simulink model "SkywalkerX8_AircraftModel"  (R2018a)
settings: Solver=FixedStepAuto  StartTime=0.0  StopTime=60  FixedStep=0.001  RelTol=1e-3
undefined symbols (not defined in the file): SkywalkerX8
settings Model: Creator=David  LastModifiedBy=David

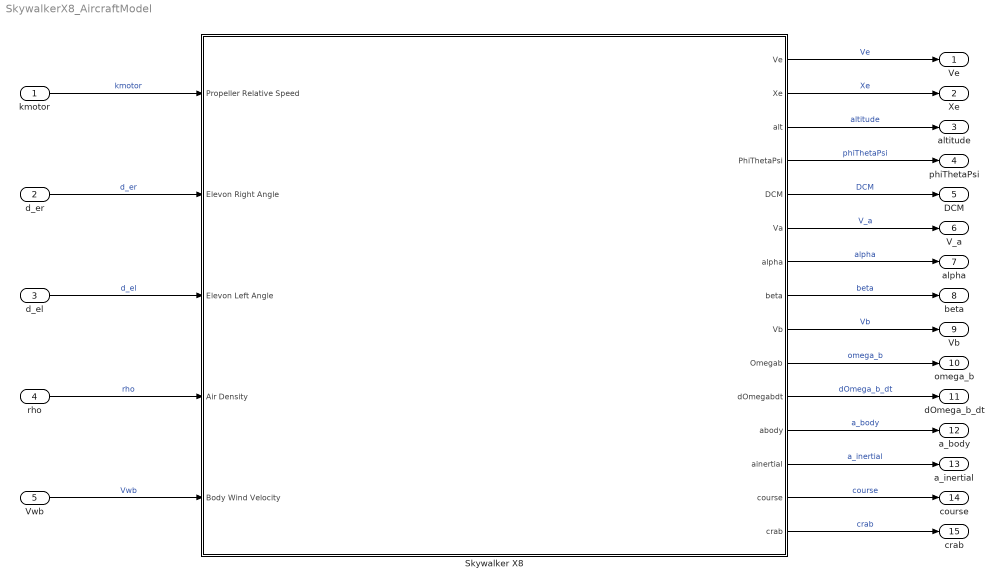
== system SkywalkerX8_AircraftModel ==
  kmotor : Inport
  d_er : Inport  Port=2
  d_el : Inport  Port=3
  rho : Inport  Port=4
  Vwb : Inport  Port=5  PortDimensions=[1, 3]
  Skywalker X8 : Subsystem  mask{PhiThetaPsi_init=[0, 0.194, 0], Xe_init=[0, 0, -100], Vb_init=[8.82, 0, 1.73], PhiThetaPsiDot_init=[0, 0, 0], Mass=SkywalkerX8.System.Mass, Inertia_Matrix=SkywalkerX8.System.InertiaTensor, g=SkywalkerX8.System.Gravity, CD=SkywalkerX8.Aerodynamics.CD, CY=SkywalkerX8.Aerodynamics.CY, CL=SkywalkerX8.Aerodynamics.CL, CI=SkywalkerX8.Aerodynamics.Cl, Cm=SkywalkerX8.Aerodynamics.Cm, Cn=SkywalkerX8.Aerodynamics.Cn, alpha_0=SkywalkerX8.Aerodynamics.alpha_0, M_trans=SkywalkerX8.Aerodynamics.M, Cmfp=SkywalkerX8.Aerodynamics.Cmfp, b=SkywalkerX8.Geometry.b, c=SkywalkerX8.Geometry.c, S=SkywalkerX8.Geometry.S, Sprop=SkywalkerX8.Propeller.Sprop, Cprop=SkywalkerX8.Propeller.Cprop, kmotor=SkywalkerX8.Propeller.kmotor, kOmega=SkywalkerX8.Propeller.kOmega, kTp=SkywalkerX8.Propeller.kTp}
      mask prompts: PhiThetaPsi_init "Inital roll, pitch and yaw angles [phi, theta, psi] (rad)"; Xe_init "Initial position in inertial frame [Xe, Ye, Ze] (m)"; Vb_init "Initial velocity in body frame [u, v, w] (m/s)"; PhiThetaPsiDot_init "Initial roll, pitch, yaw angular velocity d/dt[phi, theta, psi] (rad/s)"; Mass "System mass (kg)"; Inertia_Matrix "System Inertia Tensor [Jxx, Jxy, Jxz; Jyx, Jyy, Jyz; Jzx, Jzy, Jzz] (kg.m^2)"; g "Gravitational constant (m/s^2)"; CD "Drag force coefficient array, of multiple [1, alpha, alpha^2, cq/2Va, beta^2, beta, de^2]"; CY "Side force coefficient array, of multiple [1, beta, bp/2Va, br/2Va, da]"; CL "Lift force coefficient array, of multiple [1, alpha, cq/2Va, de]"; CI "Roll coefficient array, of multiple [1, beta, bp/2Va, br/2Va, da]"; Cm "Pitch coefficient array, of multiple [1, alpha, bq/2Va, de]"; Cn "Yaw coefficient array, of multiple [1, beta, bp/2Va, br/2Va, da]"; alpha_0 "Stall angle, alpha_0 (rad)"; M_trans "Transition rate, M"; Cmfp "Pitching moment flat plate coefficient, Cmfp"; b "Wing span, b (m)"; c "Mean aerodynamic chord, c (m)"; S "Wing area, S (m^2)"; Sprop "Propeller swept area, Sprop (m^2)"; Cprop "Propeller aerodynamic coefficient, Cprop"; kmotor "Motor constant, kmotor (m/s)"; kOmega "Motor angular velocity constant, kOmega (rad/s)"; kTp "Motor torque constant, kTp (Nm/(rad/s)^2)"
      mask DialogControl DescGroupVar Prompt: SkywalkerX8 Aircraft Model
      mask DialogControl DescTextVar Prompt: This block models the Skywalker X8 Blended Wing-Body aircraft. It takes in control inputs and environmental conditions and outputs the full 6 DoF response from the system.
      mask DialogControl Container4 Prompt: Initial Conditions
      mask DialogControl Container5 Prompt: System Characteristics
      mask DialogControl Container6 Prompt: Aerodynamic Coefficients
      mask DialogControl Container9 Prompt: Aerodynamic Stall Parameters
      mask DialogControl Container7 Prompt: Geometric Characteristics
      mask DialogControl Container10 Prompt: Propeller/Motor Characteristics
      mask Display:
      | image('C:\MATLAB\masters\icons\Skywalker Main Block Icon.png', 'center')
      | 
      | color('cyan')
      | 
      | port_label('input', 1, 'k_{motor} (Unitless)', 'texmode', 'on')
      | port_label('input', 2, '\delta_{er} (rad)', 'texmode', 'on')
      | port_label('input', 3, '\delta_{el} (rad)', 'texmode', 'on')
      | port_label('input', 4, '\rho (kg/m^3)', 'texmode', 'on')
      | port_label('input', 5, '{\bf V_w^b} (m/s)', 'texmode', 'on')
      | 
      | port_label('output', 1, '{\bf V_e} (m/s)', 'texmode', 'on')
      | port_label('output', 2, '{\bf X_e} (m)', 'texmode', 'on')
      | port_label('output', 3, 'Altitude (m)', 'texmode', 'on')
      | port_label('output', 4, '\phi \theta \psi (rad)', 'texmode', 'on')
      | port_label('output', 5, 'R_{inertial}^{body}', 'texmode', 'on')
      | port_label('output', 6, 'V_a (m/s)', 'texmode', 'on')
      | port_label('output', 7, 'alpha (rad)', 'texmode', 'on')
      | port_label('output', 8, 'beta (rad)', 'texmode', 'on')
      | port_label('output', 9, '{\bf V_b} (m/s)', 'texmode', 'on')
      | port_label('output', 10, '{\bf \omega_b} (rad/s)', 'texmode', 'on')
      | port_label('output', 11, '{\bf \delta\omega_b/\deltat} (rad/s^2)', 'texmode', 'on')
      | port_label('output', 12, '{\bf a_{body}} (m/s^2)', 'texmode', 'on')
      | port_label('output', 13, '{\bf a_{inertial}} (m/s^2)', 'texmode', 'on')
      | port_label('output', 14, '\chi (rad)', 'texmode', 'on')
      | port_label('output', 15, '\chi_c (rad)', 'texmode', 'on')
  Ve : Outport
  Xe : Outport  Port=2
  altitude : Outport  Port=3
  phiThetaPsi : Outport  Port=4
  DCM : Outport  Port=5
  V_a : Outport  Port=6
  alpha : Outport  Port=7
  beta : Outport  Port=8
  Vb : Outport  Port=9
  omega_b : Outport  Port=10
  dOmega_b_dt : Outport  Port=11
  a_body : Outport  Port=12
  a_inertial : Outport  Port=13
  course : Outport  Port=14
  crab : Outport  Port=15
  wires:
  kmotor/1 -> Skywalker X8/1(Propeller Relative Speed)  "kmotor"
  d_er/1 -> Skywalker X8/2(Elevon Right Angle)  "d_er"
  d_el/1 -> Skywalker X8/3(Elevon Left Angle)  "d_el"
  Skywalker X8/1(Ve) -> Ve/1  "Ve"
  Skywalker X8/2(Xe) -> Xe/1  "Xe"
  Skywalker X8/4(PhiThetaPsi) -> phiThetaPsi/1  "phiThetaPsi"
  Skywalker X8/9(Vb) -> Vb/1  "Vb"
  Skywalker X8/10(Omegab) -> omega_b/1  "omega_b"
  Skywalker X8/11(dOmegabdt) -> dOmega_b_dt/1  "dOmega_b_dt"
  Skywalker X8/12(abody) -> a_body/1  "a_body"
  Skywalker X8/13(ainertial) -> a_inertial/1  "a_inertial"
  rho/1 -> Skywalker X8/4(Air Density)  "rho"
  Vwb/1 -> Skywalker X8/5(Body Wind Velocity)  "Vwb"
  Skywalker X8/5(DCM) -> DCM/1  "DCM"
  Skywalker X8/6(Va) -> V_a/1  "V_a"
  Skywalker X8/3("alt ") -> altitude/1  "altitude"
  Skywalker X8/7(alpha) -> alpha/1  "alpha"
  Skywalker X8/8(beta) -> beta/1  "beta"
  Skywalker X8/14(course) -> course/1  "course"
  Skywalker X8/15(crab) -> crab/1  "crab"

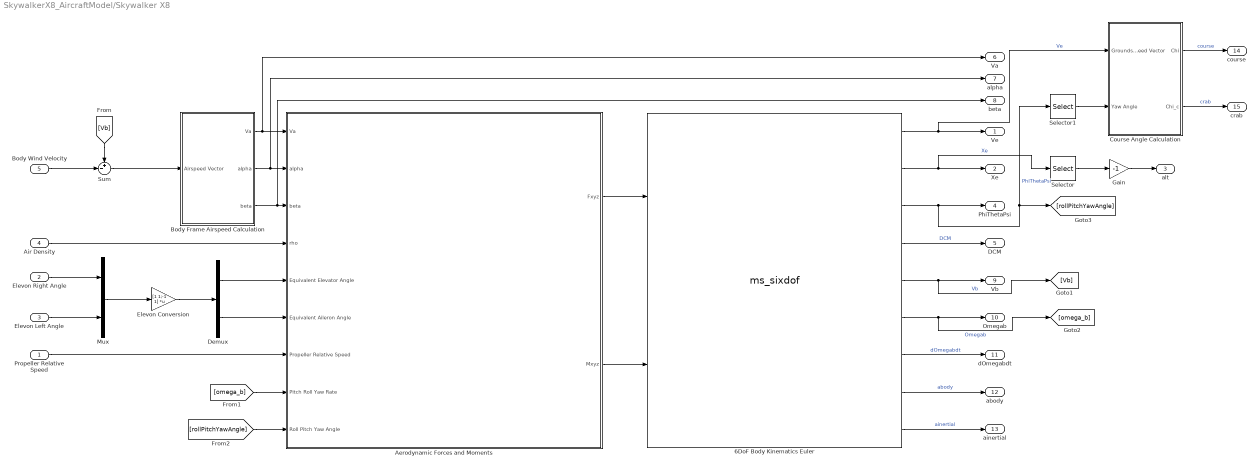
== system SkywalkerX8_AircraftModel/Skywalker X8 ==
  Propeller Relative Speed : Inport
  Elevon Right Angle : Inport  Port=2
  Elevon Left Angle : Inport  Port=3
  Air Density : Inport  Port=4
  Body Wind Velocity : Inport  Port=5
  6DoF Body Kinematics Euler : M-S-Function  FunctionName=ms_sixdof  Parameters=Xe_init, Vb_init, PhiThetaPsi_init, PhiThetaPsiDot_init, Mass, Inertia_Matrix  mask{PhiThetaPsi_init=PhiThetaPsi_init, Xe_init=Xe_init, Vb_init=Vb_init, PhiThetaPsiDot_init=PhiThetaPsiDot_init, Mass=Mass, Inertia_Matrix=Inertia_Matrix}
      mask prompts: PhiThetaPsi_init "Inital roll, pitch and yaw angles [phi, theta, psi] (rad)"; Xe_init "Initial position in inertial frame [Xe, Ye, Ze] (m)"; Vb_init "Initial velocity in body frame [u, v, w] (m/s)"; PhiThetaPsiDot_init "Initial roll, pitch, yaw angular velocity d/dt[phi, theta, psi] (rad/s)"; Mass "System mass (kg)"; Inertia_Matrix "System Inertia Tensor [Jxx, Jxy, Jxz; Jyx, Jyy, Jyz; Jzx, Jzy, Jzz] (kg.m^2)"
      mask DialogControl DescGroupVar Prompt: 6DoF Kinematics Model
      mask DialogControl DescTextVar Prompt: This block models the equations of motion for a 6DoF system in the body frame
      mask DialogControl Container4 Prompt: Initial Conditions
      mask DialogControl Container8 Prompt: System Parameters
      mask Display:
      | image('C:\MATLAB\masters\icons\6DoF Kinematics Block Icon.PNG', 'center')
      | 
      | port_label('input', 1, '{\bf F_{xyz}} (N)', 'texmode', 'on')
      | port_label('input', 2, '{\bf M_{xyz}} (Nm)', 'texmode', 'on')
      | 
      | port_label('output', 1, '{\bf V_e} (m/s)', 'texmode', 'on')
      | port_label('output', 2, '{\bf X_e} (m)', 'texmode', 'on')
      | port_label('output', 3, '\phi \theta \psi (rad)', 'texmode', 'on')
      | port_label('output', 4, 'R_{inertial}^{body}', 'texmode', 'on')
      | port_label('output', 5, '{\bf V_b} (m/s)', 'texmode', 'on')
      | port_label('output', 6, '{\bf \omega_b} (rad/s)', 'texmode', 'on')
      | port_label('output', 7, '{\bf \delta\omega_b/\deltat} (rad/s^2)', 'texmode', 'on')
      | port_label('output', 8, '{\bf a_{body}} (m/s^2)', 'texmode', 'on')
      | port_label('output', 9, '{\bf a_{inertial}} (m/s^2)', 'texmode', 'on')
  Aerodynamic Forces and Moments : Subsystem  mask{CD=CD, CY=CY, CL=CL, CI=CI, Cm=Cm, Cn=Cn, alpha_0=alpha_0, M_trans=M_trans, Cmfp=Cmfp, b=b, c=c, S=S, m=Mass, g=g, Sprop=Sprop, Cprop=Cprop, kmotor=kmotor, kOmega=kOmega, kTp=kTp}
      mask prompts: CD "Drag force coefficient array, of multiple [1, alpha, alpha^2, cq/2Va, beta^2, beta, de^2]"; CY "Side force coefficient array, of multiple [1, beta, bp/2Va, br/2Va, da]"; CL "Lift force coefficient array, of multiple [1, alpha, cq/2Va, de]"; CI "Roll coefficient array, of multiple [1, beta, bp/2Va, br/2Va, da]"; Cm "Pitch coefficient array, of multiple [1, alpha, bq/2Va, de]"; Cn "Yaw coefficient array, of multiple [1, beta, bp/2Va, br/2Va, da]"; alpha_0 "Stall angle, alpha_0 (rad)"; M_trans "Transition rate, M"; Cmfp "Pitching moment flat plate coefficient, Cmfp"; b "Wing span, b (m)"; c "Mean aerodynamic chord, c (m)"; S "Wing area, S (m^2)"; m "System mass, m (kg)"; g "Gravitational constant, g (m/s^2)"; Sprop "Propeller swept area, Sprop (m^2)"; Cprop "Propeller aerodynamic coefficient, Cprop"; kmotor "Motor constant, kmotor (m/s)"; kOmega "Motor angular velocity constant, kOmega (rad/s)"; kTp "Motor torque constant, kTp (Nm/(rad/s)^2)"
      mask DialogControl DescGroupVar Prompt: Aerodynamic Forces and Moments
      mask DialogControl DescTextVar Prompt: The purpose of this block is to calulate the aerodynamic forces and moments expeirenced by an aircraft exposed to a particular airflow, at a particular density, given a particular set of control surface inputs and motor parameters. This will also depend on the systems current state in terms of body rotational velocity and angles.
      mask DialogControl Container4 Prompt: Aerodynamic Coeffecients
      mask DialogControl Container10 Prompt: Aerodynamic Stall Parameters
      mask DialogControl Container5 Prompt: Geometric Characteristics
      mask DialogControl Container6 Prompt: System Characteristics
      mask DialogControl Container7 Prompt: Propeller/Motor Characteristics
      mask Display:
      | image('C:\MATLAB\masters\icons\Skywalker Aerodynamic Block Icon.PNG', 'center')
      | 
      | port_label('input', 1, 'V_{a} (m/s)', 'texmode', 'on')
      | port_label('input', 2, '\alpha (rad)', 'texmode', 'on')
      | port_label('input', 3, '\beta (rad)', 'texmode', 'on')
      | port_label('input', 4, '\rho (kg/m^3)', 'texmode', 'on')
      | port_label('input', 5, '\delta_e (rad)', 'texmode', 'on')
      | port_label('input', 6, '\delta_a (rad)', 'texmode', 'on')
      | port_label('input', 7, '\delta_{t} (Unitless)', 'texmode', 'on')
      | port_label('input', 8, '{\bf\omega_b} (rad/s)', 'texmode', 'on')
      | port_label('input', 9, '\phi \theta \psi (rad)', 'texmode', 'on')
      | 
      | port_label('output', 1, '{\bf F_{xyz}} (N)', 'texmode', 'on')
      | port_label('output', 2, '{\bf M_{xyz}} (Nm)', 'texmode', 'on')
  Body Frame Airspeed Calculation : Subsystem
      mask Display:
      | port_label('input', 1, '{\bf V_{a}^{b}} (m/s)', 'texmode', 'on')
      | 
      | port_label('output', 1, 'V_{a} (m/s)', 'texmode', 'on')
      | port_label('output', 2, '\alpha (rad)', 'texmode', 'on')
      | port_label('output', 3, '\beta (rad)', 'texmode', 'on')
  Course Angle Calculation : Subsystem
      mask Display:
      | port_label('input', 1, '{\bf V_{e}} (m/s)', 'texmode', 'on')
      | port_label('input', 2, '\psi (rad)', 'texmode', 'on')
      | 
      | port_label('output', 1, '\chi (rad)', 'texmode', 'on')
      | port_label('output', 2, '\chi_c (rad)', 'texmode', 'on')
  Demux : Demux  Outputs=2
  Elevon Conversion : Gain  Gain=[1 1;-1 1]  Multiplication=Matrix(K*u)
  Gain : Gain  Gain=-1
  Mux : Mux  Inputs=2
  Selector : Selector  InputPortWidth=3  IndexOptions=Index vector (dialog)  Indices=3  OutputSizes=1
  Selector1 : Selector  InputPortWidth=3  IndexOptions=Index vector (dialog)  Indices=3  OutputSizes=1
  Sum : Sum  Inputs=+-|
  Ve : Outport
  Xe : Outport  Port=2
  "alt " : Outport  Port=3
  PhiThetaPsi : Outport  Port=4
  DCM : Outport  Port=5
  Va : Outport  Port=6
  alpha : Outport  Port=7
  beta : Outport  Port=8
  Vb : Outport  Port=9
  Omegab : Outport  Port=10
  dOmegabdt : Outport  Port=11
  abody : Outport  Port=12
  ainertial : Outport  Port=13
  course : Outport  Port=14
  crab : Outport  Port=15
  wires:
  Elevon Left Angle/1 -> Mux/2
  6DoF Body Kinematics Euler/8 -> abody/1  "abody"
  Elevon Conversion/1 -> Demux/1
  6DoF Body Kinematics Euler/2 -> Xe/1, Selector/1  "Xe"
  6DoF Body Kinematics Euler/1 -> Ve/1, Course Angle Calculation/1(Groundspeed Vector)  "Ve"
  [rollPitchYawAngle] -> Aerodynamic Forces and Moments/9("Roll Pitch Yaw Angle ")
  Mux/1 -> Elevon Conversion/1
  Elevon Right Angle/1 -> Mux/1
  Air Density/1 -> Aerodynamic Forces and Moments/4(rho)
  Body Frame Airspeed Calculation/2(alpha) -> alpha/1, Aerodynamic Forces and Moments/2(alpha)
  Body Wind Velocity/1 -> Sum/2
  Body Frame Airspeed Calculation/1(Va) -> Aerodynamic Forces and Moments/1(Va), Va/1
  Demux/2 -> Aerodynamic Forces and Moments/6(Equivalent Aileron Angle)
  6DoF Body Kinematics Euler/7 -> dOmegabdt/1  "dOmegabdt"
  Body Frame Airspeed Calculation/3(beta) -> beta/1, Aerodynamic Forces and Moments/3(beta)
  [Vb] -> Sum/1
  Demux/1 -> Aerodynamic Forces and Moments/5(Equivalent Elevator Angle)
  Propeller Relative Speed/1 -> Aerodynamic Forces and Moments/7(Propeller Relative Speed)
  [omega_b] -> Aerodynamic Forces and Moments/8(Pitch Roll Yaw Rate)
  Sum/1 -> Body Frame Airspeed Calculation/1(Airspeed Vector)
  6DoF Body Kinematics Euler/9 -> ainertial/1  "ainertial"
  6DoF Body Kinematics Euler/3 -> Selector1/1, [rollPitchYawAngle], PhiThetaPsi/1  "PhiThetaPsi"
  6DoF Body Kinematics Euler/4 -> DCM/1  "DCM"
  6DoF Body Kinematics Euler/5 -> [Vb], Vb/1  "Vb"
  6DoF Body Kinematics Euler/6 -> [omega_b], Omegab/1  "Omegab"
  Aerodynamic Forces and Moments/2(Mxyz) -> 6DoF Body Kinematics Euler/2
  Aerodynamic Forces and Moments/1(Fxyz) -> 6DoF Body Kinematics Euler/1
  Selector/1 -> Gain/1
  Gain/1 -> "alt "/1
  Selector1/1 -> Course Angle Calculation/2(Yaw Angle)
  Course Angle Calculation/1(Chi) -> course/1  "course"
  Course Angle Calculation/2(Chi_c) -> crab/1  "crab"

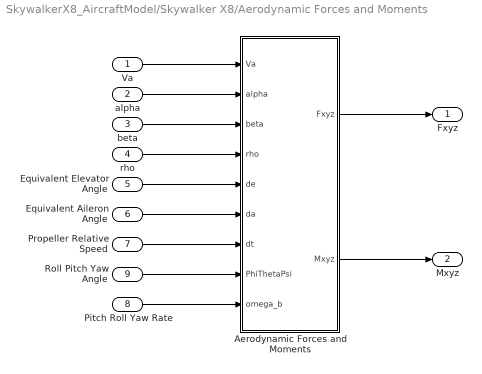
== system SkywalkerX8_AircraftModel/Skywalker X8/Aerodynamic Forces and Moments ==
  Va : Inport
  alpha : Inport  Port=2
  beta : Inport  Port=3
  rho : Inport  Port=4
  Equivalent Elevator Angle : Inport  Port=5
  Equivalent Aileron Angle : Inport  Port=6
  Propeller Relative Speed : Inport  Port=7
  Pitch Roll Yaw Rate : Inport  Port=8
  "Roll Pitch Yaw Angle " : Inport  Port=9
  Aerodynamic Forces and Moments : MATLAB Function  TreatAsAtomicUnit=on
  Fxyz : Outport
  Mxyz : Outport  Port=2
  wires:
  Aerodynamic Forces and Moments/1(Fxyz) -> Fxyz/1
  Aerodynamic Forces and Moments/2(Mxyz) -> Mxyz/1
  Va/1 -> Aerodynamic Forces and Moments/1(Va)
  alpha/1 -> Aerodynamic Forces and Moments/2(alpha)
  beta/1 -> Aerodynamic Forces and Moments/3(beta)
  rho/1 -> Aerodynamic Forces and Moments/4(rho)
  Equivalent Elevator Angle/1 -> Aerodynamic Forces and Moments/5(de)
  Equivalent Aileron Angle/1 -> Aerodynamic Forces and Moments/6(da)
  Pitch Roll Yaw Rate/1 -> Aerodynamic Forces and Moments/9(omega_b)
  "Roll Pitch Yaw Angle "/1 -> Aerodynamic Forces and Moments/8(PhiThetaPsi)
  Propeller Relative Speed/1 -> Aerodynamic Forces and Moments/7(dt)

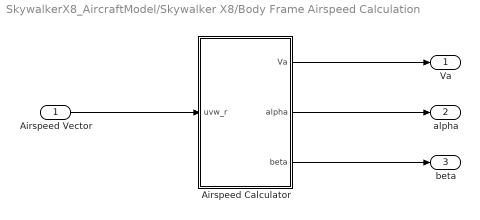
== system SkywalkerX8_AircraftModel/Skywalker X8/Body Frame Airspeed Calculation ==
  Airspeed Vector : Inport
  Airspeed Calculator : MATLAB Function  TreatAsAtomicUnit=on
  Va : Outport
  alpha : Outport  Port=2
  beta : Outport  Port=3
  wires:
  Airspeed Vector/1 -> Airspeed Calculator/1(uvw_r)
  Airspeed Calculator/1(Va) -> Va/1
  Airspeed Calculator/2(alpha) -> alpha/1
  Airspeed Calculator/3(beta) -> beta/1

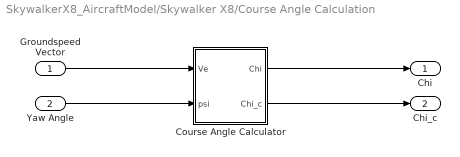
== system SkywalkerX8_AircraftModel/Skywalker X8/Course Angle Calculation ==
  Groundspeed Vector : Inport
  Yaw Angle : Inport  Port=2
  Course Angle Calculator : MATLAB Function  TreatAsAtomicUnit=on
  Chi : Outport
  Chi_c : Outport  Port=2
  wires:
  Groundspeed Vector/1 -> Course Angle Calculator/1(Ve)
  Course Angle Calculator/1(Chi) -> Chi/1
  Course Angle Calculator/2(Chi_c) -> Chi_c/1
  Yaw Angle/1 -> Course Angle Calculator/2(psi)

== matlab function SkywalkerX8_AircraftModel/Skywalker X8/Aerodynamic Forces and Moments/Aerodynamic Forces and Moments ==
  data: Va input; Fxyz output; alpha input; beta input; rho input; de input; da input; dt input; PhiThetaPsi input; Mxyz output; omega_b input; CD parameter; CY parameter; CL parameter; CI parameter; Cm parameter; Cn parameter; m parameter; g parameter; S parameter; b parameter; c parameter; Sprop parameter; Cprop parameter; kmotor parameter; kTp parameter; kOmega parameter; Cmfp parameter; M_trans parameter; alpha_0 parameter
function [Fxyz, Mxyz] = fcn(Va, alpha, beta, rho, de, da, dt, PhiThetaPsi, omega_b, CD, CY, CL, CI, Cm, Cn, m, g, S, b, c, Sprop, Cprop, kmotor, kTp, kOmega, Cmfp, M_trans, alpha_0)

[Fxyz, Mxyz] = f_ForcesAndMoments(Va, alpha, beta, rho, de, da, dt, PhiThetaPsi, omega_b, CD, CY, CL, CI, Cm, Cn, m, g, S, b, c, Sprop, Cprop, kmotor, kTp, kOmega, Cmfp, M_trans, alpha_0);

end

== matlab function SkywalkerX8_AircraftModel/Skywalker X8/Body Frame Airspeed Calculation/Airspeed Calculator ==
  data: uvw_r input; Va output; alpha output; beta output
 function [Va, alpha, beta] = fcn(uvw_r)

    Va = sqrt(uvw_r*uvw_r');
    
    alpha = atan2(uvw_r(3), uvw_r(1));
    
    if (Va ~= 0)
        
        beta = asin(uvw_r(2)/Va);
    
    else
        
        beta = 0;
        
    end
end

== matlab function SkywalkerX8_AircraftModel/Skywalker X8/Course Angle Calculation/Course Angle Calculator ==
  data: Ve input; Chi output; psi input; Chi_c output
function [Chi, Chi_c] = fcn(Ve, psi)

Chi = atan2(Ve(1), Ve(2));
Chi_c = Chi - psi;
